simulink model "attitudeSensors"  (R2023b)
settings: Solver=VariableStepAuto  StartTime=0.0  StopTime=Tfinal  RelTol=1e-3
model workspace: external: MAT-File starTrackerSimpleUndersampled.mat (data not in the file)
undefined symbols (not defined in the file or in its folder): attitudeNoiseFactor, Vstar, wstar
libraries: matrix_library x1, sensorToolsLib x1
settings Model: Creator=kristopherriordan  LastModifiedBy=kristopherriordan

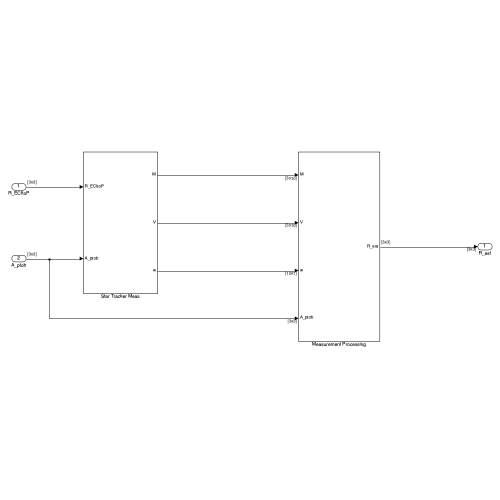
[thumbnail: Simulink's stored preview of the top-level diagram]
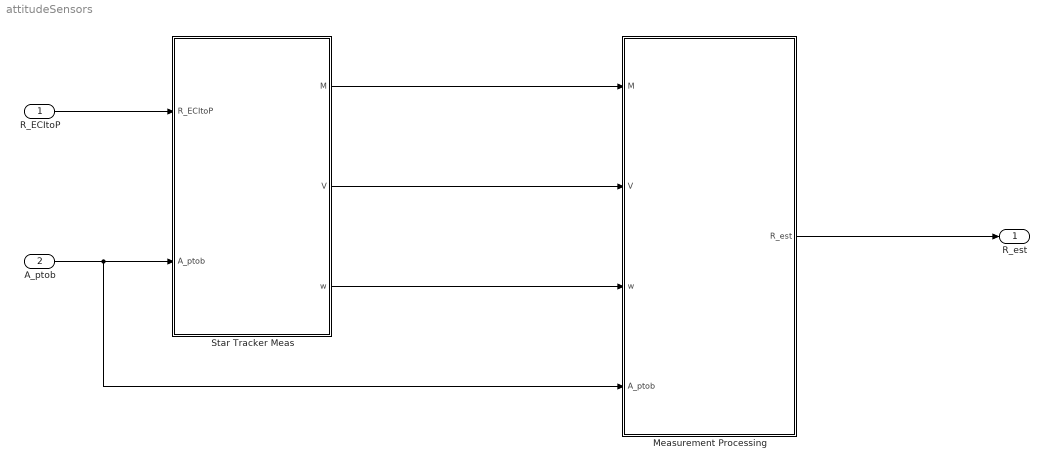
== system attitudeSensors ==
  R_ECItoP : Inport  PortDimensions=[3 3]
  A_ptob : Inport  Port=2  PortDimensions=[3 3]
  Measurement Processing : Subsystem
  Star Tracker Meas : Subsystem
  R_est : Outport  PortDimensions=[3 3]
  wires:
  R_ECItoP/1 -> Star Tracker Meas/1(R_ECItoP)
  A_ptob/1 -> Measurement Processing/4(A_ptob), Star Tracker Meas/2(A_ptob)
  Star Tracker Meas/1(M) -> Measurement Processing/1(M)
  Star Tracker Meas/2(V) -> Measurement Processing/2(V)
  Star Tracker Meas/3(w) -> Measurement Processing/3(w)
  Measurement Processing/1(R_est) -> R_est/1

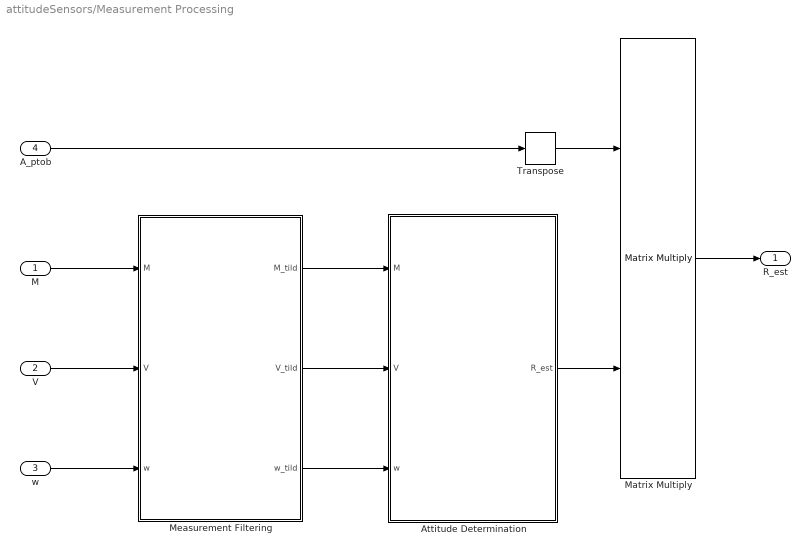
== system attitudeSensors/Measurement Processing ==
  M : Inport  PortDimensions=size(Vstar)
  V : Inport  Port=2  PortDimensions=size(Vstar)
  w : Inport  Port=3  PortDimensions=size(wstar)
  A_ptob : Inport  Port=4  PortDimensions=[3 3]
  Attitude Determination : Subsystem  Variant=on
  Matrix Multiply : Product  Multiplication=Matrix(*)
  Measurement Filtering : Subsystem
  Transpose : matrix_library/Transpose
  R_est : Outport  PortDimensions=[3 3]
  wires:
  V/1 -> Measurement Filtering/2(V)
  M/1 -> Measurement Filtering/1(M)
  Measurement Filtering/1(M_tild) -> Attitude Determination/1(M)
  Measurement Filtering/2(V_tild) -> Attitude Determination/2(V)
  Measurement Filtering/3(w_tild) -> Attitude Determination/3(w)
  w/1 -> Measurement Filtering/3(w)
  A_ptob/1 -> Transpose/1
  Attitude Determination/1(R_est) -> Matrix Multiply/2
  Transpose/1 -> Matrix Multiply/1
  Matrix Multiply/1 -> R_est/1

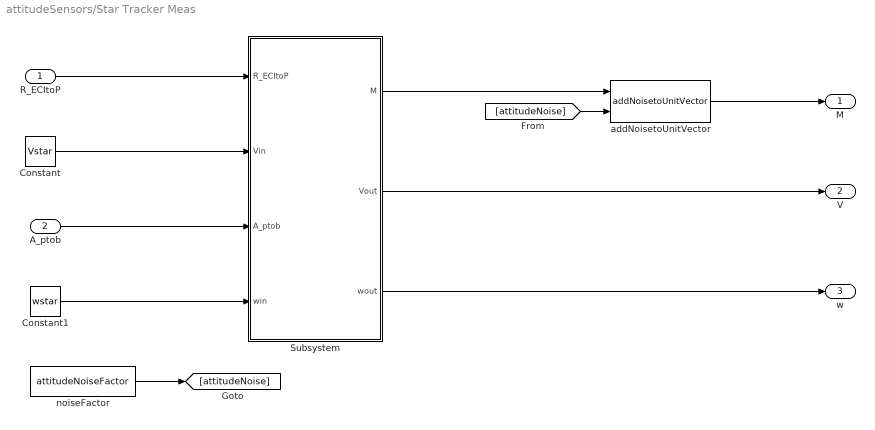
== system attitudeSensors/Star Tracker Meas ==
  R_ECItoP : Inport
  A_ptob : Inport  Port=2
  Constant : Constant  Value=Vstar  VectorParams1D=off
  Constant1 : Constant  Value=wstar  VectorParams1D=off
  Subsystem : Subsystem  Variant=on  VariantControlMode=label  VariantControl=Subsystem  LabelModeActiveChoice="starCatalog==\"simple\""
  addNoisetoUnitVector : sensorToolsLib/addNoisetoUnitVector  SystemSampleTime=-1  VariantActivationTime=update diagram  AllowFlexibleInterface=on  Latency=0  AutoFrameSizeCalculation=off
  noiseFactor : Constant  Value=attitudeNoiseFactor
  M : Outport
  V : Outport  Port=2
  w : Outport  Port=3
  wires:
  R_ECItoP/1 -> Subsystem/1(R_ECItoP)
  Constant/1 -> Subsystem/2(Vin)
  A_ptob/1 -> Subsystem/3(A_ptob)
  Constant1/1 -> Subsystem/4(win)
  Subsystem/1(M) -> addNoisetoUnitVector/1
  Subsystem/2(Vout) -> V/1
  Subsystem/3(wout) -> w/1
  noiseFactor/1 -> [attitudeNoise]
  [attitudeNoise] -> addNoisetoUnitVector/2
  addNoisetoUnitVector/1 -> M/1

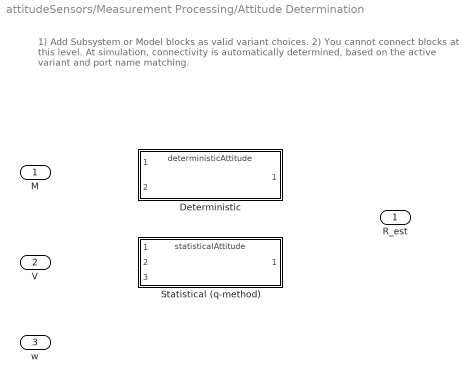
== system attitudeSensors/Measurement Processing/Attitude Determination ==
  note: 1) Add Subsystem or Model blocks as valid variant choices.
      | 2) You cannot connect blocks at this level. At simulation, connectivity is automatically
      | determined, based on the active variant and port name matching.
  M : Inport
  V : Inport  Port=2
  w : Inport  Port=3
  Deterministic : ModelReference  ModelNameDialog=deterministicAttitude.slx  SimulationMode=Normal  VariantControl="attitudeSensorSolver==\"deterministic\""  ModelReferenceVersion=1.9
  Statistical (q-method) : ModelReference  ModelNameDialog=statisticalAttitude.slx  SimulationMode=Normal  VariantControl="attitudeSensorSolver==\"qmethod\""  ModelReferenceVersion=1.7
  R_est : Outport  PortDimensions=[3 3]

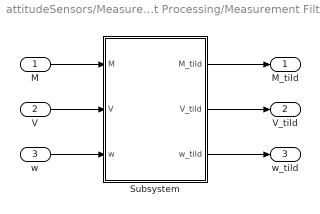
== system attitudeSensors/Measurement Processing/Measurement Filtering ==
  M : Inport
  V : Inport  Port=2
  w : Inport  Port=3
  Subsystem : Subsystem  Variant=on  VariantControl=Subsystem
  M_tild : Outport
  V_tild : Outport  Port=2
  w_tild : Outport  Port=3
  wires:
  M/1 -> Subsystem/1(M)
  V/1 -> Subsystem/2(V)
  w/1 -> Subsystem/3(w)
  Subsystem/1(M_tild) -> M_tild/1
  Subsystem/2(V_tild) -> V_tild/1
  Subsystem/3(w_tild) -> w_tild/1

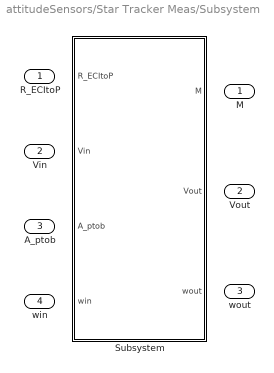
== system attitudeSensors/Star Tracker Meas/Subsystem ==
  R_ECItoP : Inport
  Vin : Inport  Port=2
  A_ptob : Inport  Port=3
  win : Inport  Port=4
  Subsystem : Subsystem  VariantControl="starCatalog==\"simple\""
  M : Outport
  Vout : Outport  Port=2
  wout : Outport  Port=3

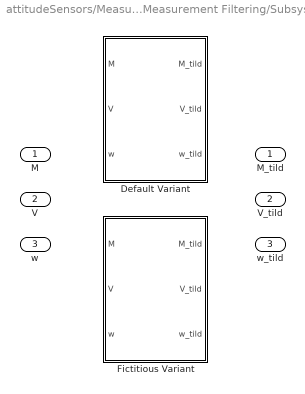
== system attitudeSensors/Measurement Processing/Measurement Filtering/Subsystem ==
  M : Inport
  V : Inport  Port=2
  w : Inport  Port=3
  "Default Variant " : Subsystem  VariantControl="measProcess==\"default\""
  Fictitious Variant : Subsystem  VariantControl="measProcess==\"fictitious\""
  M_tild : Outport
  V_tild : Outport  Port=2
  w_tild : Outport  Port=3

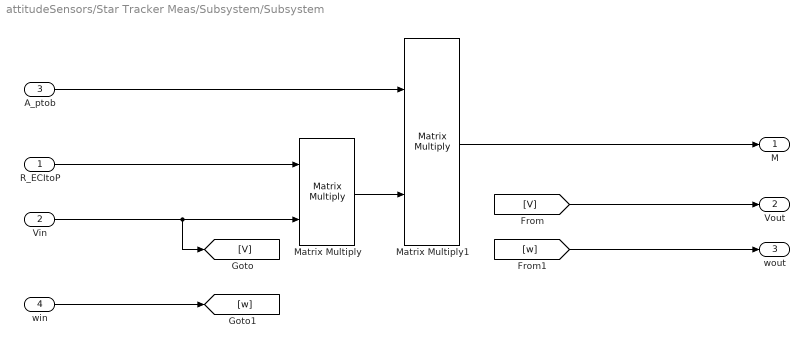
== system attitudeSensors/Star Tracker Meas/Subsystem/Subsystem ==
  R_ECItoP : Inport
  Vin : Inport  Port=2
  A_ptob : Inport  Port=3
  win : Inport  Port=4
  Matrix Multiply : Product  Multiplication=Matrix(*)
  Matrix Multiply1 : Product  Multiplication=Matrix(*)
  M : Outport
  Vout : Outport  Port=2
  wout : Outport  Port=3
  wires:
  A_ptob/1 -> Matrix Multiply1/1
  R_ECItoP/1 -> Matrix Multiply/1
  [V] -> Vout/1
  [w] -> wout/1
  win/1 -> [w]
  Vin/1 -> Matrix Multiply/2, [V]
  Matrix Multiply1/1 -> M/1
  Matrix Multiply/1 -> Matrix Multiply1/2

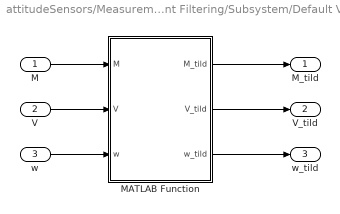
== system attitudeSensors/Measurement Processing/Measurement Filtering/Subsystem/Default Variant  ==
  M : Inport
  V : Inport  Port=2
  w : Inport  Port=3
  MATLAB Function : MATLAB Function  TreatAsAtomicUnit=on
  M_tild : Outport
  V_tild : Outport  Port=2
  w_tild : Outport  Port=3
  wires:
  MATLAB Function/3(w_tild) -> w_tild/1
  V/1 -> MATLAB Function/2(V)
  w/1 -> MATLAB Function/3(w)
  MATLAB Function/2(V_tild) -> V_tild/1
  MATLAB Function/1(M_tild) -> M_tild/1
  M/1 -> MATLAB Function/1(M)

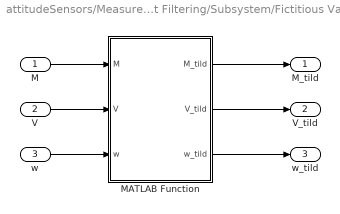
== system attitudeSensors/Measurement Processing/Measurement Filtering/Subsystem/Fictitious Variant ==
  M : Inport
  V : Inport  Port=2
  w : Inport  Port=3
  MATLAB Function : MATLAB Function  TreatAsAtomicUnit=on
  M_tild : Outport
  V_tild : Outport  Port=2
  w_tild : Outport  Port=3
  wires:
  MATLAB Function/3(w_tild) -> w_tild/1
  V/1 -> MATLAB Function/2(V)
  w/1 -> MATLAB Function/3(w)
  MATLAB Function/2(V_tild) -> V_tild/1
  MATLAB Function/1(M_tild) -> M_tild/1
  M/1 -> MATLAB Function/1(M)

== matlab function attitudeSensors/Measurement Processing/Measurement Filtering/Subsystem/Default Variant /MATLAB Function ==
  data: M input; M_tild output; V input; w input; V_tild output; w_tild output
function [M_tild,V_tild, w_tild] = defaultMeasVariant(M, V, w)

n = size(M, 2);

if n > 2
    M_tild = M;
    V_tild = V;
    w_tild = w;
elseif n == 2
    m1_int = M(:,1);
    m2_int = M(:,2);

    v1_int = V(:,1);
    v2_int = V(:,2);
    
    pm = m1_int;
    qm = cross(m1_int, m2_int)./norm(cross(m1_int, m2_int));
    rm = cross(pm, qm);

    pv = v1_int;
    qv = cross(v1_int, v2_int)./norm(cross(v1_int, v2_int));
    rv = cross(pv, qv);
    
    M_tild = [pm, qm, rm];
    V_tild = [pv, qv, rv];
    w_tild = [w; min(w)];
end

== matlab function attitudeSensors/Measurement Processing/Measurement Filtering/Subsystem/Fictitious Variant/MATLAB Function ==
  data: M input; M_tild output; V input; w input; V_tild output; w_tild output
function [M_tild,V_tild, w_tild] = fictitiousMeasVariant(M, V, w)

n = size(M, 2);

if n > 2
    M_tild = M;
    V_tild = V;
    w_tild = w;
elseif n == 2
    m1_int = (M(:,1) + M(:,2))./2;
    m2_int = (M(:,1) - M(:,2))./2;

    v1_int = (V(:,1) + V(:,2))./2;
    v2_int = (V(:,1) - V(:,2))./2;
    
    pm = m1_int;
    qm = cross(m1_int, m2_int)./norm(cross(m1_int, m2_int));
    rm = cross(pm, qm);

    pv = v1_int;
    qv = cross(v1_int, v2_int)./norm(cross(v1_int, v2_int));
    rv = cross(pv, qv);
    
    M_tild = [pm, qm, rm];
    V_tild = [pv, qv, rv];
    w_tild = ones([3 1]);
end
